simulink model "Assignment_1__Two_spring_mass_damper"  (R2019b)
settings: Solver=VariableStepAuto  StartTime=0.0  StopTime=10.0  RelTol=1e-3
undefined symbols (not defined in the file): c1, c2, k1, k2, m1, m2
libraries: simulink x1
settings Model: Creator=Vishrant  LastModifiedBy=Vishrant

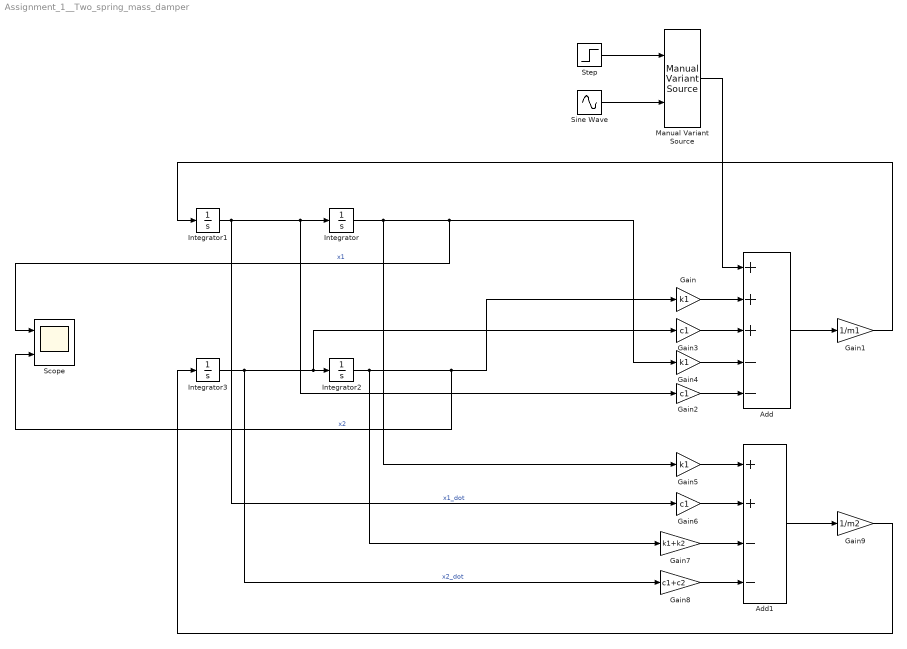
== system Assignment_1__Two_spring_mass_damper ==
  Add : Sum  Inputs=+++--
  Add1 : Sum  Inputs=++--
  Gain : Gain  Gain=k1
  Gain1 : Gain  Gain=1/m1
  Gain2 : Gain  Gain=c1
  Gain3 : Gain  Gain=c1
  Gain4 : Gain  Gain=k1
  Gain5 : Gain  Gain=k1
  Gain6 : Gain  Gain=c1
  Gain7 : Gain  Gain=k1+k2
  Gain8 : Gain  Gain=c1+c2
  Gain9 : Gain  Gain=1/m2
  Integrator{,1..3} (4 alike) : Integrator
  Manual Variant Source : simulink/Signal Routing/Manual Variant Source  NumChoices=2  LabelModeActiveChoice=V_1
      settings: SourceProductName=Simulink
  Scope : Scope  NumInputPorts=2
  Sine Wave : Sin  Amplitude=3  Frequency=10  SampleTime=0
  Step : Step  After=5  SampleTime=0
  wires:
  Integrator/1 -> Gain5/1, Scope/1, Gain4/1  "x1"
  Integrator1/1 -> Gain6/1, Gain2/1, Integrator/1  "x1_dot"
  Integrator3/1 -> Gain8/1, Gain3/1, Integrator2/1  "x2_dot"
  Integrator2/1 -> Gain7/1, Scope/2, Gain/1  "x2"
  Gain/1 -> Add/2
  Gain3/1 -> Add/3
  Gain4/1 -> Add/4
  Gain2/1 -> Add/5
  Add/1 -> Gain1/1
  Gain1/1 -> Integrator1/1
  Gain5/1 -> Add1/1
  Gain6/1 -> Add1/2
  Gain7/1 -> Add1/3
  Gain8/1 -> Add1/4
  Gain9/1 -> Integrator3/1
  Add1/1 -> Gain9/1
  Sine Wave/1 -> Manual Variant Source/2
  Manual Variant Source/1 -> Add/1
  Step/1 -> Manual Variant Source/1
